simulink model "SinglePhaseInverter"  (R2018a)
settings: Solver=ode23s  StartTime=0  StopTime=totalSim  FixedStep=StepTime  MaxStep=StepTime  EnableMultiTasking=on
values from neighbouring files (symbols this model uses):
  C = 20e-6    (= 2e-05)    [SinglePhaseInverterData.m]
  f1 = 50*2*pi    (= 314.159265359)    [SinglePhaseInverterData.m]
  L = 100e-3    (= 0.1)    [SinglePhaseInverterData.m]
  ma = 0.8    [SinglePhaseInverterData.m]
  Modo = 1    [SinglePhaseInverterData.m]
  Rload = 78.26    [SinglePhaseInverterData.m]
  Ts = 1/Fs    (= 0.000333333333333)    [SinglePhaseInverterData.m]
  vcc = 100    [SinglePhaseInverterData.m]
libraries: powerlib x14, simulink x1
settings Model: Creator=fl4862  LastModifiedBy=facu
settings DataIOCC: LimitDataPoints=on  SaveFormat=Array  SignalLoggingSaveFormat=ModelDataLogs
settings OptimizationCC: ExpressionDepthLimit=2147483647  LifeSpan=inf
settings DebuggingCC: UnderspecifiedInitializationDetection=Classic  MergeDetectMultiDrivingBlocksExec=none  SolverPrmCheckMsg=warning  FcnCallInpInsideContextMsg=warning  StateNameClashWarn=warning  LibraryContextMissingDiagnostic=warning  SFUnexpectedBacktrackingDiag=warning  SFNoUnconditionalDefaultTransitionDiag=warning  SFExecutionAtInitializationDiag=none
settings HardwareCC: ProdBitPerPointer=32  ProdBitPerSizeT=32  ProdBitPerPtrDiffT=32  ProdLargestAtomicFloat=None  ProdIntDivRoundTo=Undefined  ProdEndianess=Unspecified  ProdWordSize=32  ProdHWDeviceType=32-bit Generic
settings ModelReferenceCC: PropagateSignalLabelsOutOfModel=off
settings CodeAppCC: StateflowObjectComments=on
settings GRTTargetCC: TargetLangStandard=C89/C90 (ANSI)  GeneratePreprocessorConditionals=Disable all  CombineOutputUpdateFcns=off  GRTInterface=on
settings ConfigComp: CovMetricSettings=dw  CovHtmlReporting=on  CovSaveCumulativeToWorkspaceVar=on  CovSaveSingleToWorkspaceVar=on  CovExternalEMLEnable=off  CovSFcnEnable=off
settings SimscapeCC: SimscapeNormalizeSystem=off

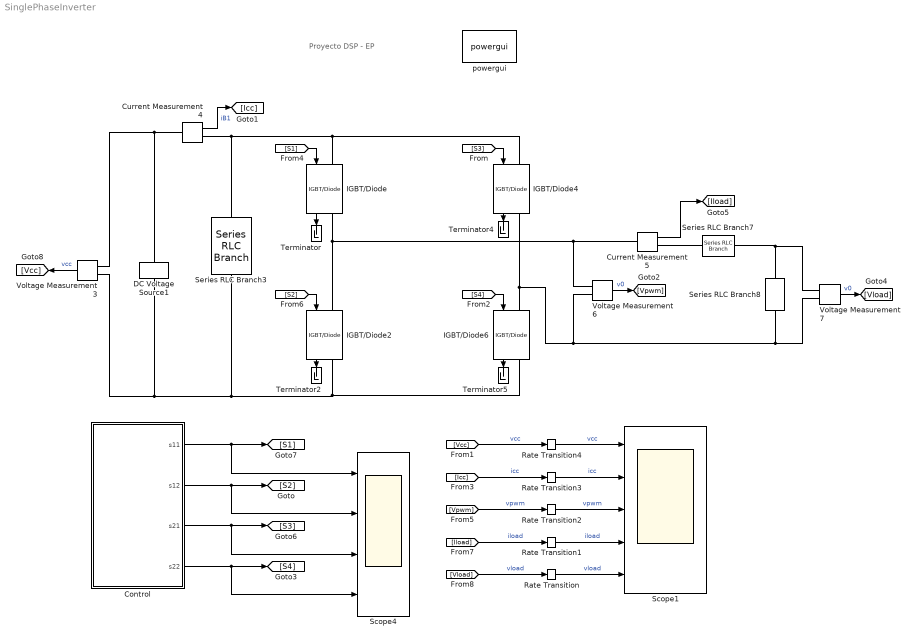
== system SinglePhaseInverter ==
  note: Proyecto DSP - EP
  Control : Subsystem
  Current Measurement4 : powerlib/Measurements/Current Measurement  PhasorSimulation=off  OutputType=Complex  PSBequivalent=0
  Current Measurement5 : powerlib/Measurements/Current Measurement  PhasorSimulation=off  OutputType=Complex  PSBequivalent=0
  DC Voltage Source1 : powerlib/Electrical Sources/DC Voltage Source  Amplitude=vcc  Measurements=None
  IGBT/Diode{,2,4,6} (4 alike) : powerlib/Power Electronics/IGBT//Diode  Ron=1e-7  Rs=1e5  Cs=inf  Measurements=on
  Rate Transition{,1..4} (5 alike) : RateTransition  OutPortSampleTime=Tsample
  Scope1 : Scope  NumInputPorts=5
  Scope4 : Scope  NumInputPorts=4
  Series RLC Branch3 : powerlib/Elements/Series RLC Branch  LConnTagsString=__new0  RConnTagsString=__new0  BranchType=RC  Resistance=1e-9  Inductance=1e-3  SetiL0=off  InitialCurrent=0  Capacitance=C  Setx0=on  InitialVoltage=vcc  Measurements=None
  Series RLC Branch7 : powerlib/Elements/Series RLC Branch  LConnTagsString=__new0  RConnTagsString=__new0  BranchType=L  Resistance=1  Inductance=L  SetiL0=on  InitialCurrent=0  Capacitance=1e-6  Setx0=off  InitialVoltage=0  Measurements=None
  Series RLC Branch8 : powerlib/Elements/Series RLC Branch  LConnTagsString=__new0  RConnTagsString=__new0  BranchType=R  Resistance=Rload  Inductance=L  SetiL0=on  InitialCurrent=0  Capacitance=1e-6  Setx0=off  InitialVoltage=0  Measurements=None
  Terminator{,2,4..5} (4 alike) : Terminator
  Voltage Measurement3 : powerlib/Measurements/Voltage Measurement  PhasorSimulation=off  OutputType=Complex  PSBequivalent=0
  Voltage Measurement6 : powerlib/Measurements/Voltage Measurement  PhasorSimulation=off  OutputType=Complex  PSBequivalent=0
  Voltage Measurement7 : powerlib/Measurements/Voltage Measurement  PhasorSimulation=off  OutputType=Complex  PSBequivalent=0
  powergui : powerlib/powergui  Priority=1  SimulationMode=Continuous  SampleTime=50e-6  frequency=60  Iterations=50  frequencyindice=0  Pbase=100e6  ErrMax=1e-4  UnitsV=kV  UnitsW=MW  buscounter=0  FunctionMessages=off  echomessages=off  EnableUseOfTLC=off  CurrentSourceSwitches=off  DisableSnubberDevices=off  DisableRonSwitches=off  DisableVfSwitches=off  DisplayEquations=off  SolverType=Tustin  Interpol=off  ExternalGateDelay=off  methode=off  Ts=0  x0status=blocks  SPID=off  SwTol=0  HookPort=off  RestoreLinks=warning  ResistiveCurrentMeasurement=off  Frange=[0:2:500]  Ylog=off  Xlog=on  ShowGrid=off  save=off  variable=ZData  structure=0  ZoomFFT=off  StartTime=0.0  cycles=1  DisplayStyle=1  fundamental=60  FreqAxis=off  MaxFrequency=1000  frequencyindicesteady=1  RmsSteady=1  display=off
  wires:
  [S2] -> IGBT/Diode2/1
  [S1] -> IGBT/Diode/1
  IGBT/Diode2/1 -> Terminator2/1
  IGBT/Diode/1 -> Terminator/1
  Voltage Measurement3/1 -> [Vcc]  "vcc"
  Control/1(s11) -> [S1], Scope4/1
  Control/2(s12) -> [S2], Scope4/2
  Control/3(s21) -> [S3], Scope4/3
  Control/4(s22) -> [S4], Scope4/4
  IGBT/Diode4/1 -> Terminator4/1
  [S4] -> IGBT/Diode6/1
  IGBT/Diode6/1 -> Terminator5/1
  [S3] -> IGBT/Diode4/1
  Current Measurement4/1 -> [Icc]  "iB1"
  Voltage Measurement6/1 -> [Vpwm]  "v0"
  Voltage Measurement7/1 -> [Vload]  "v0"
  Current Measurement5/1 -> [Iload]
  [Vcc] -> Rate Transition4/1  "vcc"
  [Icc] -> Rate Transition3/1  "icc"
  [Vpwm] -> Rate Transition2/1  "vpwm"
  [Iload] -> Rate Transition1/1  "iload"
  [Vload] -> Rate Transition/1  "vload"
  Rate Transition/1 -> Scope1/5  "vload"
  Rate Transition1/1 -> Scope1/4  "iload"
  Rate Transition3/1 -> Scope1/2  "icc"
  Rate Transition2/1 -> Scope1/3  "vpwm"
  Rate Transition4/1 -> Scope1/1  "vcc"
  connections:
  IGBT/Diode6/RConn1 -- IGBT/Diode2/RConn1 -- Series RLC Branch3/RConn1 -- DC Voltage Source1/LConn1 -- Voltage Measurement3/LConn2
  Series RLC Branch3/LConn1 -- IGBT/Diode4/LConn1 -- IGBT/Diode/LConn1 -- Current Measurement4/RConn1
  IGBT/Diode/RConn1 -- Voltage Measurement6/LConn1 -- Current Measurement5/LConn1 -- IGBT/Diode2/LConn1
  Voltage Measurement3/LConn1 -- DC Voltage Source1/RConn1 -- Current Measurement4/LConn1
  IGBT/Diode4/RConn1 -- Voltage Measurement7/LConn2 -- Series RLC Branch8/RConn1 -- Voltage Measurement6/LConn2 -- IGBT/Diode6/LConn1
  Series RLC Branch7/RConn1 -- Voltage Measurement7/LConn1 -- Series RLC Branch8/LConn1
  Current Measurement5/RConn1 -- Series RLC Branch7/LConn1

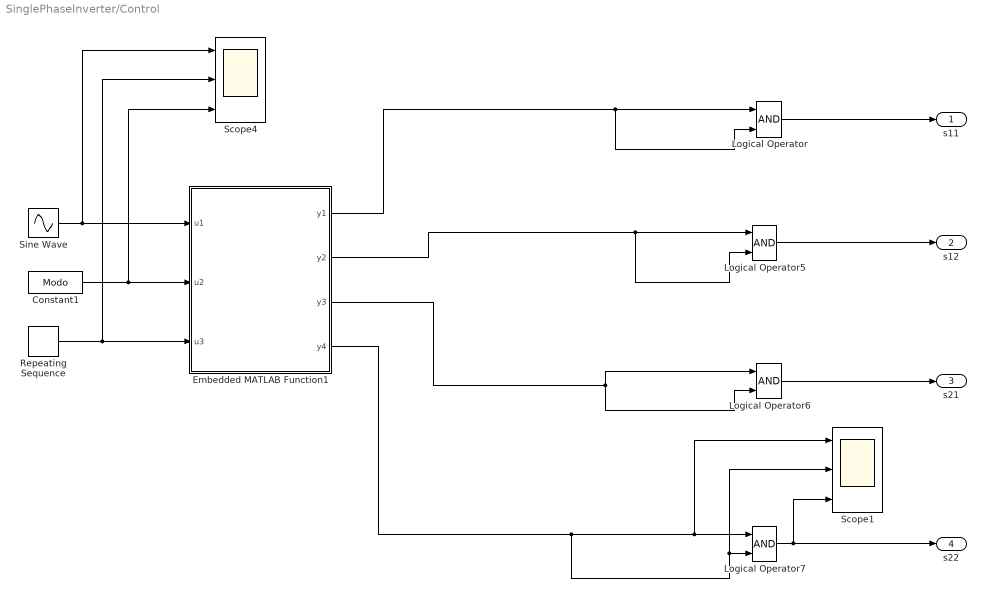
== system SinglePhaseInverter/Control ==
  Constant1 : Constant  Value=Modo
  Embedded MATLAB Function1 : MATLAB Function  TreatAsAtomicUnit=on
  Logical Operator{,5..7} (4 alike) : Logic  IconShape=distinctive  AllPortsSameDT=off  OutDataTypeStr=boolean
  Repeating Sequence : simulink/Sources/Repeating Sequence  rep_seq_t=[0 Ts/2 Ts]  rep_seq_y=[-1 1 -1]
  Scope1 : Scope  NumInputPorts=3
  Scope4 : Scope  NumInputPorts=3
  Sine Wave : Sin  Amplitude=ma  Frequency=f1  SampleTime=0
  s11 : Outport
  s12 : Outport  Port=2
  s21 : Outport  Port=3
  s22 : Outport  Port=4
  wires:
  Embedded MATLAB Function1/1(y1) -> Logical Operator/2, Logical Operator/1
  Embedded MATLAB Function1/2(y2) -> Logical Operator5/2, Logical Operator5/1
  Embedded MATLAB Function1/3(y3) -> Logical Operator6/2, Logical Operator6/1
  Logical Operator/1 -> s11/1
  Logical Operator5/1 -> s12/1
  Logical Operator6/1 -> s21/1
  Logical Operator7/1 -> s22/1, Scope1/3
  Sine Wave/1 -> Scope4/1, Embedded MATLAB Function1/1(u1)
  Constant1/1 -> Embedded MATLAB Function1/2(u2), Scope4/3
  Embedded MATLAB Function1/4(y4) -> Logical Operator7/2, Scope1/2, Logical Operator7/1, Scope1/1
  Repeating Sequence/1 -> Scope4/2, Embedded MATLAB Function1/3(u3)

== matlab function SinglePhaseInverter/Control/Embedded MATLAB Function1 ==
  data: u1 input; y1 output; u2 input; u3 input; y2 output; y3 output; y4 output
function [y1,y2,y3,y4] = fcn(u1,u2,u3)
% This block supports the Embedded MATLAB subset.
% See the help menu for details. 

mode = round(u2);

if(mode == 1) % Buck Continuous mode
    
    if(u1 >= u3)
        y1 = 1;
        y2 = 0;
        
        y3 = y2;
        y4 = y1;
        
    else
        y1 = 0;
        y2 = 1;
        
        y3 = y2;
        y4 = y1;
    
    end
    
elseif(mode == 2)

    if(u1 >= u3)
        y1 = 1;
        y2 = 0;
        
    else
        y1 = 0;
        y2 = 1;
        
    end
    
    if(-u1 < u3)
        y4 = 1;
        y3 = 0;
        
    else
        y4 = 0;
        y3 = 1;
        
    end
    
else
    
    y1 = 0;
    y2 = 0;
    y3 = 0;
    y4 = 0;
    
end
